simulink model "AEBfinal"  (R2023b)
settings: Solver=FixedStepAuto  StartTime=0.0  StopTime=inf  FixedStep=0.01  RelTol=1e-3
libraries: motar_bsw_lib x6
settings Model: DataDictionary=AEBfinal_MotarConfig.sldd  Creator=20221261  LastModifiedBy=20221261
settings OptimizationCC: DefaultParameterBehavior=Inlined  EnhancedBackFolding=on  PassReuseOutputArgsAs=Individual arguments  ZeroExternalMemoryAtStartup=off  ZeroInternalMemoryAtStartup=off  NoFixptDivByZeroProtection=on  EfficientFloat2IntCast=on  OptimizeBlockOrder=speed  DifferentSizesBufferReuse=on  OptimizationCustomize=off  EfficientTunableParamExpr=on
settings DebuggingCC: ParameterTunabilityLossMsg=error
settings HardwareCC: ProdBitPerPointer=32  ProdBitPerSizeT=32  ProdBitPerPtrDiffT=32  ProdLargestAtomicInteger=Long  ProdLargestAtomicFloat=Double  ProdEndianess=BigEndian  ProdWordSize=32  ProdHWDeviceType=TTTech->TTC 500
settings SFSimCC: MATLABDynamicMemAlloc=off
settings RTWCC: Description=ICT Motar Dx  SystemTargetFile=Motar_Dx.tlc  EmbeddedCoderDictionary=AEBfinal_MotarConfig.sldd  TemplateMakefile=Motar_Dx.tmf  GenerateReport=on  LaunchReport=on
settings RTWCC: CustomHeaderCode=|
  | /* Function prototypes for safeRTOS */
  | #ifdef EXT_MODE
  | #include "rtos_tasks.h"
  | /* Main function task for RTOS*/
  | int main_init(ttc_task_init_struct_t init_data);
  | void main_cyclic(void);
  | #endif /* EXT_MODE */
settings CodeAppCC: ForceParamTrailComments=on  IgnoreCustomStorageClasses=off  MaxIdLength=255  OperatorAnnotations=on  SimulinkDataObjDesc=on  SFDataObjDesc=on  InsertBlockDesc=on
settings STFCustomTargetCC: TargetLibSuffix=.a  MultiwordLength=256  CompOptLevelCompliant=on  IncludeMdlTerminateFcn=off  CombineOutputUpdateFcns=on  ERTCustomFileBanners=on  SupportContinuousTime=off  RemoveResetFunc=on  MATLABClassNameForMDSCustomization=Simulink.SoftwareTarget.ERTCustomization  SystemTargetFile=Motar_Dx.tlc
settings ERTTargetCC: TargetLangStandard=C99 (ISO)  ParMdlRefBuildCompliant=off  ConcurrentExecutionCompliant=off  IncludeMdlTerminateFcn=off  SupportNonInlinedSFcns=on  ModelStepFunctionPrototypeControlCompliant=off  CPPClassGenCompliant=off  UseToolchainInfoCompliant=off  InlinedParameterPlacement=NonHierarchical  ERTCustomFileTemplate=Dx_file_process.tlc  MemSecPackage=tms570ls31  MemSecDataConstants=MPU1_DATA_START  MemSecDataIO=MPU1_DATA_START  MemSecDataInternal=MPU1_DATA_START  MemSecDataParameters=MPU1_DATA_START  MemSecFuncInitTerm=MPU1_DATA_START

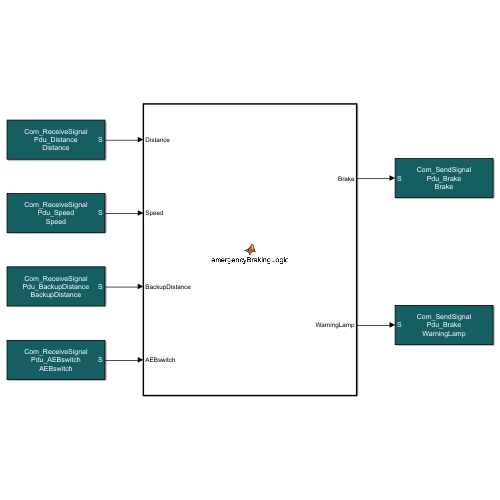
[thumbnail: Simulink's stored preview of the top-level diagram]
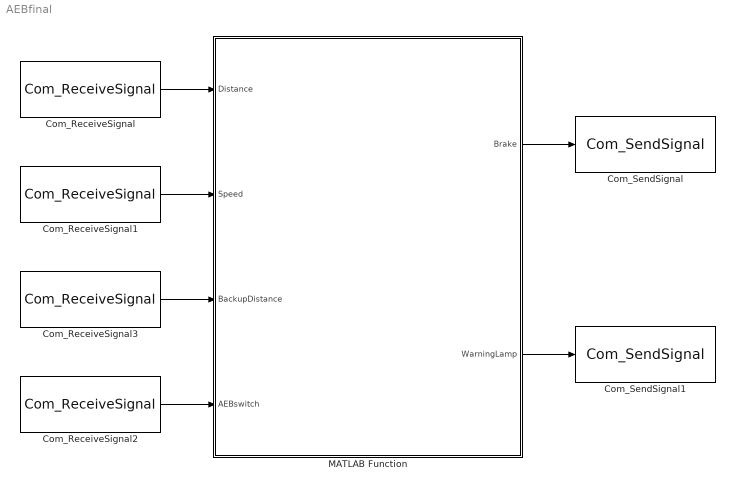
== system AEBfinal ==
  Com_ReceiveSignal : motar_bsw_lib/ComStack/Com_ReceiveSignal  PduName=char('Pdu_Distance')  SignalName=char('Distance')  SignalSize=uint32(8)  SignalWidth=uint32(1)  SignalTimeout=uint32(0)  ChosenOption=uint8(0)  inputConstant=char('0')  inputMATLAB=char('inputMATLAB.m')  tsamp=0.01
      settings: SourceProductName=ICT Motar Toolbox
  Com_ReceiveSignal1 : motar_bsw_lib/ComStack/Com_ReceiveSignal  PduName=char('Pdu_Speed')  SignalName=char('Speed')  SignalSize=uint32(8)  SignalWidth=uint32(1)  SignalTimeout=uint32(0)  ChosenOption=uint8(0)  inputConstant=char('0')  inputMATLAB=char('inputMATLAB.m')  tsamp=0.01
      settings: SourceProductName=ICT Motar Toolbox
  Com_ReceiveSignal2 : motar_bsw_lib/ComStack/Com_ReceiveSignal  PduName=char('Pdu_AEBswitch')  SignalName=char('AEBswitch')  SignalSize=uint32(8)  SignalWidth=uint32(1)  SignalTimeout=uint32(0)  ChosenOption=uint8(0)  inputConstant=char('0')  inputMATLAB=char('inputMATLAB.m')  tsamp=0.01
      settings: SourceProductName=ICT Motar Toolbox
  Com_ReceiveSignal3 : motar_bsw_lib/ComStack/Com_ReceiveSignal  PduName=char('Pdu_BackupDistance')  SignalName=char('BackupDistance')  SignalSize=uint32(8)  SignalWidth=uint32(1)  SignalTimeout=uint32(0)  ChosenOption=uint8(0)  inputConstant=char('0')  inputMATLAB=char('inputMATLAB.m')  tsamp=0.01
      settings: SourceProductName=ICT Motar Toolbox
  Com_SendSignal : motar_bsw_lib/ComStack/Com_SendSignal  PduName=char('Pdu_Brake')  SignalName=char('Brake')  SignalSize=uint32(8)  SignalWidth=uint32(1)  tsamp=-1
      settings: SourceProductName=ICT Motar Toolbox
  Com_SendSignal1 : motar_bsw_lib/ComStack/Com_SendSignal  PduName=char('Pdu_Brake')  SignalName=char('WarningLamp')  SignalSize=uint32(8)  SignalWidth=uint32(1)  tsamp=-1
      settings: SourceProductName=ICT Motar Toolbox
  MATLAB Function : MATLAB Function  TreatAsAtomicUnit=on
  wires:
  Com_ReceiveSignal/1 -> MATLAB Function/1(Distance)
  MATLAB Function/1(Brake) -> Com_SendSignal/1
  Com_ReceiveSignal1/1 -> MATLAB Function/2(Speed)
  Com_ReceiveSignal2/1 -> MATLAB Function/4(AEBswitch)
  MATLAB Function/2(WarningLamp) -> Com_SendSignal1/1
  Com_ReceiveSignal3/1 -> MATLAB Function/3(BackupDistance)

== matlab function AEBfinal/MATLAB Function ==
  data: Distance input; Brake output; Speed input; BackupDistance input; AEBswitch input; WarningLamp output
function [Brake, WarningLamp] = emergencyBrakingLogic(Distance, Speed, BackupDistance, AEBswitch)
% EMERGENCYBRAKINGLOGIC Calculate brake intensity based on filtered distance
% Distance: Smoothed distance data (single)
% Speed: Vehicle speed in kmph (uint8)
% BackupDistance: Backup distance input in case primary fails (uint8)
% AEBswitch: Automatic Emergency Braking switch (1 for ON, 0 for OFF)
% Brake: Braking intensity as a value from 0 to 100 (uint8)
% WarningLamp: Warning signal output (1 if primary sensor fails, 0 otherwise)
persistent brake_history brake_active threshold_set Distance_threshold min_distance;
window_size = 300; % Larger window size for even smoother results (adjustable)
% Initialize persistent variables
if isempty(brake_history)
    brake_history = single(zeros(window_size, 1));
    brake_active = false; % Flag to indicate if brake should stay fully on
    threshold_set = false; % Flag to check if threshold has been set based on initial distance check
    Distance_threshold = single(20); % Default threshold to 20 if speed <= 55
    min_distance = single(12); % Minimum distance for full braking application
end
% Initialize output values
Brake = uint8(0);
WarningLamp = uint8(0); % Default to 0, indicating no warning
% Convert Distance and BackupDistance from uint8 to single for calculations
Distance = single(Distance);
BackupDistance = single(BackupDistance);
max_Brake = single(100); % Maximum brake intensity (0 to 100)
% Check if primary Distance data is valid (non-zero and received)
if Distance <= 0
    % If primary distance is invalid, switch to backup and activate warning
    Distance = BackupDistance;
    WarningLamp = uint8(1); % Set warning signal to 1
end
% Reset brake if AEB is switched off
if AEBswitch == 0
    brake_active = false; % Reset the brake active flag when AEB is off
    Brake = uint8(0); % No brake when AEB is off
    WarningLamp = uint8(1); % Set warning signal to 1
    threshold_set = false; % Reset threshold check
    Distance_threshold = single(20); % Reset to default threshold
    min_distance = single(12); % Reset to default minimum distance
    return;
end
% Check distance and set threshold based on speed when distance drops below 22 for the first time
if Distance < 22 && ~threshold_set
    if Speed > 55
        Distance_threshold = single(22); % Set threshold to 22 if speed > 55
        min_distance = single(20); % Set minimum distance to 20 if speed > 55
    else
        Distance_threshold = single(20); % Set threshold to 20 if speed <= 55
        min_distance = single(12); % Set minimum distance to 12 if speed <= 55
    end
    threshold_set = true; % Threshold set, so do not reset
end
% Braking logic
% Once the distance is below min_distance, brake remains fully engaged
if Distance <= min_distance && Speed > 10
    brake_active = true; % Activate the brake persistence when distance is below min_distance
end
% If the brake is active, keep it fully engaged
if brake_active
    Brake = uint8(100); % Keep brake fully applied
    return; % No further calculations needed
end
% Normal braking logic before the distance drops below min_distance
if AEBswitch == 1
    if Distance <= Distance_threshold && Distance > min_distance
        % Linear braking response for smoother braking
        Brake_value = max_Brake * (Distance_threshold - Distance) / (Distance_threshold - min_distance);
    elseif Distance <= min_distance
        Brake_value = max_Brake;
    else
        Brake_value = single(0);
    end
    
    Brake = uint8(round(Brake_value));
end
end
